simulink model "FM_Transmitter_NBFM"  (R2022a)
settings: Solver=FixedStepDiscrete  StartTime=0.0  StopTime=inf  RelTol=1e-3
undefined symbols (not defined in the file): DiscIntNeverNeededParam
libraries: dspsrcs4 x2, simulink x1, dsparch4 x1
settings Model: Creator=vovan  LastModifiedBy=vovan

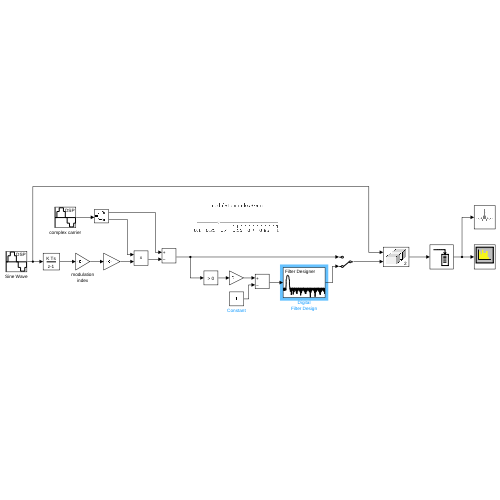
[thumbnail: Simulink's stored preview of the top-level diagram]
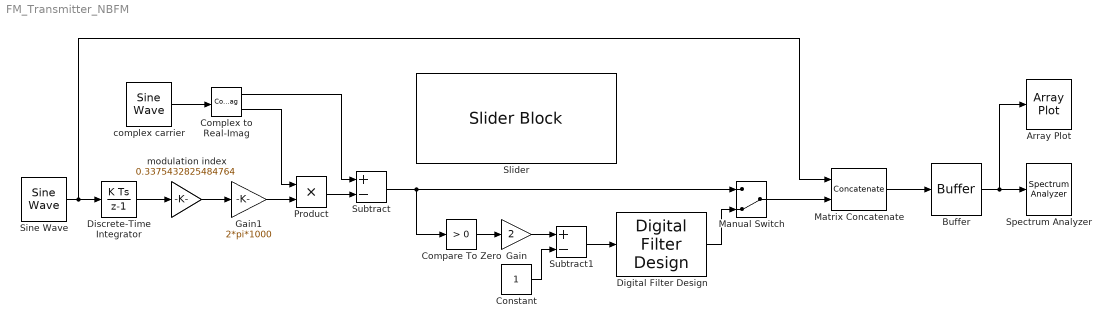
== system FM_Transmitter_NBFM ==
  Array Plot : ArrayPlot  WindowPosition=[1121.000000,6.000000,800.000000,500.000000,]  Visible=on  ScopeFrameLocation=window  PlotType=Line  YLimits=[-1.8024,1.7946]  ShowLegend=on  MeasurementChannel=2
  Buffer : Buffer  N=1024  OutputFrames=off
  Compare To Zero : simulink/Logic and Bit Operations/Compare To Zero  relop=>  OutDataTypeStr=boolean
  Complex to Real-Imag : ComplexToRealImag
  Constant : Constant
  Digital Filter Design : dsparch4/Digital Filter Design  mwdsp_browser_bugfix_var=off
  Discrete-Time Integrator : DiscreteIntegrator  SampleTime=-1  ICPrevOutput=DiscIntNeverNeededParam  ICPrevScaledInput=DiscIntNeverNeededParam
  Gain : Gain  Gain=2
  Gain1 : Gain  Gain=2*pi*1000
  Manual Switch : ManualSwitch  CurrentSetting=0
  Matrix Concatenate : Concatenate  Mode=Multidimensional array  ConcatenateDimension=2
  Product : Product
  Sine Wave : dspsrcs4/Sine Wave  Amplitude=1  Frequency=1e3  Phase=0  SampleMode=Discrete  OutComplex=Real  CompMethod=Trigonometric fcn  TableSize=Speed  SampleTime=1/200e3  SamplesPerFrame=1  ResetState=Restart at time zero  OutputFrames=off  dataType=double  wordLen=16  udDataType=sfix(16)  fracBitsMode=Best precision  numFracBits=15  OutDataTypeStr=double  LastOutDataTypeStr=double
  Slider : SliderBlock  ScaleMin=0.1  ScaleMax=1
  Spectrum Analyzer : SpectrumAnalyzer
  Subtract : Sum  Inputs=+-
  Subtract1 : Sum  Inputs=+-
  complex carrier : dspsrcs4/Sine Wave  Amplitude=1  Frequency=10e3  Phase=0  SampleMode=Discrete  OutComplex=Complex  CompMethod=Trigonometric fcn  TableSize=Speed  SampleTime=1/200e3  SamplesPerFrame=1  ResetState=Restart at time zero  OutputFrames=off  dataType=double  wordLen=16  udDataType=sfix(16)  fracBitsMode=Best precision  numFracBits=15  OutDataTypeStr=double  LastOutDataTypeStr=double
  modulation index : Gain  Gain=0.3375432825484764
  wires:
  Discrete-Time Integrator/1 -> modulation index/1
  Matrix Concatenate/1 -> Buffer/1
  complex carrier/1 -> Complex to Real-Imag/1
  modulation index/1 -> Gain1/1
  Complex to Real-Imag/2 -> Product/1
  Gain1/1 -> Product/2
  Product/1 -> Subtract/2
  Complex to Real-Imag/1 -> Subtract/1
  Sine Wave/1 -> Matrix Concatenate/1, Discrete-Time Integrator/1
  Buffer/1 -> Array Plot/1, Spectrum Analyzer/1
  Constant/1 -> Subtract1/2
  Subtract/1 -> Compare To Zero/1, Manual Switch/1
  Compare To Zero/1 -> Gain/1
  Gain/1 -> Subtract1/1
  Subtract1/1 -> Digital Filter Design/1
  Manual Switch/1 -> Matrix Concatenate/2
  Digital Filter Design/1 -> Manual Switch/2
